simulink model "ball_balancing_platform"  (R2023b)
settings: Solver=VariableStepAuto  StartTime=0.0  StopTime=10.0  RelTol=1e-3
values from neighbouring files (symbols this model uses):
  A = [0 0 0 0 0 0 0 0 0 0 0 0 ... (16 elements, 4x4)]    [LMPC.mat]    (also in ball_balancing_platform.mat = [0 0 0 0 0 0 0 0 0 0 0 0 ... (64 elements, 8x8)]; new.mat = [0 0 0 0 0 0 0 0 0 0 0 0 ... (144 elements, 12x12)])
  B = [1 0 0 0 0 1 0 0 0 0 1 0 ... (16 elements, 4x4)]    [LMPC.mat]    (also in ball_balancing_platform.mat = [0 0 0 0 0 0 1 0 0 0 0 0 ... (16 elements, 8x2)]; new.mat = [0 0 0 0 0 0 0 0 0.769230769231 0 0 0 ... (48 elements, 12x4)
  C = [1 0 0 0 0 1 0 0 0 0 1 0 ... (16 elements, 4x4)]    [LMPC.mat]    (also in ball_balancing_platform.mat = [1 0 0 0 0 1 0 0 0 0 1 0 ... (32 elements, 4x8)]; new.mat = [1 0 0 0 0 0 0 1 0 0 0 0 ... (72 elements, 6x12)])
  D = [0 0 0 0 0 0 0 0 0 0 0 0 ... (16 elements, 4x4)]    [LMPC.mat]    (also in ball_balancing_platform.mat = [0  0; 0  0; 0  0; 0  0]; new.mat = [0 0 0 0 0 0 0 0 0 0 0 0 ... (24 elements, 6x4)])
libraries: mpclib x1
settings Model: Creator=farhan  LastModifiedBy=farhan

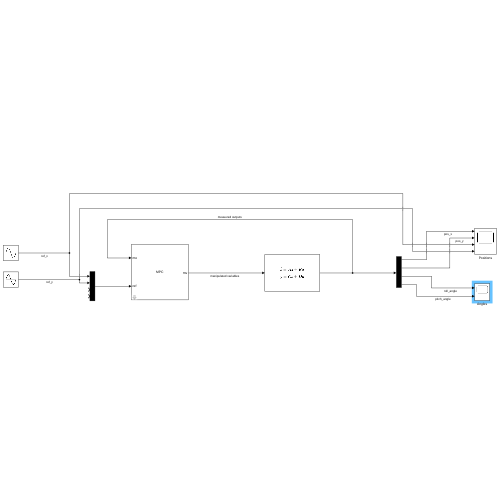
[thumbnail: Simulink's stored preview of the top-level diagram]
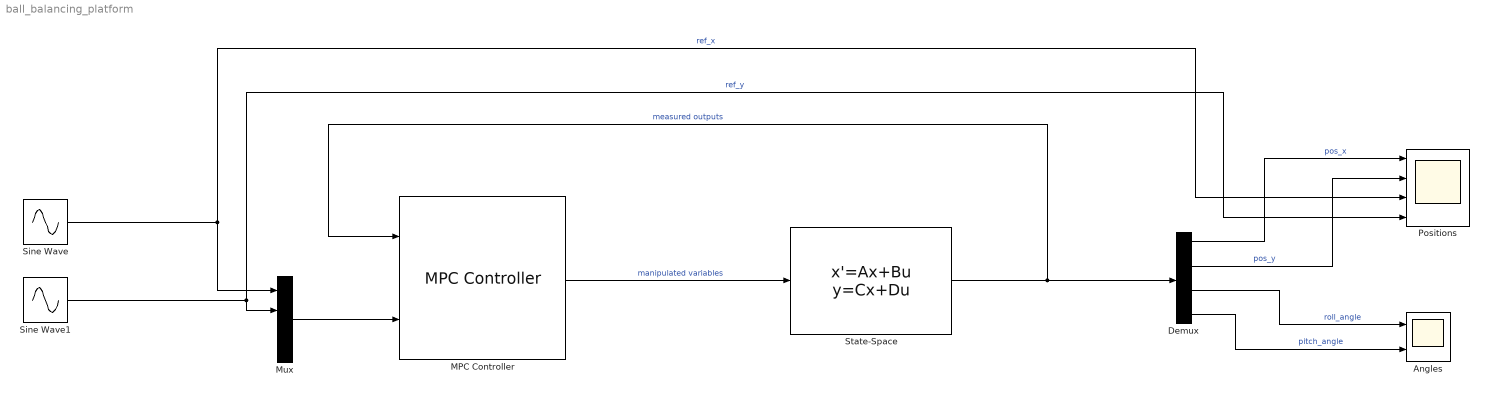
== system ball_balancing_platform ==
  Angles : Scope  NumInputPorts=2
  Demux : Demux
  MPC Controller : mpclib/MPC Controller  SCDEnableBlockLinearizationSpecification=on  mpcobj=mpc1  is_multiple=0  enable_value=0  return_u0=off  updateMPCinCallerWorkspace=on  md_inport=off  mv_inport=off  uref_inport=off  return_cost=off  return_mvseq=off  return_qpstatus=off  return_xseq=off  return_state=off  return_ovseq=off  state_inport=off  umin_inport=off  umax_inport=off  ymin_inport=off  ymax_inport=off  cc_inport=off  ywt_inport=off  uwt_inport=off  duwt_inport=off  rhoeps_inport=off  pm_inport=off  MaximumP=10  HorizonChoice=FixedHorizon  n_ts=0.1  n_p=7  n_mv=2  n_md=0  n_ud=0  n_mo=4  n_uo=0  BlockDataType=double  SampleTimeInherited=off  switch_inport=off
  Mux : Mux
  Positions : Scope  NumInputPorts=4
  Sine Wave : Sin  Amplitude=0.030  SampleTime=0
  Sine Wave1 : Sin  Amplitude=0.015  SampleTime=0
  State-Space : StateSpace  A=A  B=B  C=C  D=D  InitialCondition=0
  wires:
  MPC Controller/1 -> State-Space/1  "manipulated variables"
  State-Space/1 -> Demux/1, MPC Controller/1  "measured outputs"
  Demux/1 -> Positions/1  "pos_x"
  Demux/2 -> Positions/2  "pos_y"
  Mux/1 -> MPC Controller/2
  Demux/3 -> Angles/1  "roll_angle"
  Demux/4 -> Angles/2  "pitch_angle"
  Sine Wave/1 -> Mux/1, Positions/3  "ref_x"
  Sine Wave1/1 -> Mux/2, Positions/4  "ref_y"
